simulink model "ThurstCalculation_Part1"  (R2017b)
settings: Solver=ode2  StartTime=0.0  StopTime=10  FixedStep=1/100  RelTol=1e-3  EnableMultiTasking=on
settings Model: Creator=dsde009  LastModifiedBy=Danyck
settings SolverCC: AlgebraicLoopSolver=LineSearch
settings DataIOCC: LimitDataPoints=on  SaveFormat=Array  SignalLoggingSaveFormat=ModelDataLogs  SignalLoggingName=SPE_DataLog
settings OptimizationCC: ExpressionDepthLimit=2147483647  InitFltsAndDblsToZero=on  LifeSpan=inf
settings DebuggingCC: ReadBeforeWriteMsg=DisableAll  WriteAfterWriteMsg=DisableAll  WriteAfterReadMsg=DisableAll  AlgebraicLoopMsg=none  SaveWithDisabledLinksMsg=none  UnderspecifiedInitializationDetection=Classic  MergeDetectMultiDrivingBlocksExec=none  MultiTaskDSMMsg=warning  MultiTaskCondExecSysMsg=none  ParameterPrecisionLossMsg=none  StateNameClashWarn=warning  SFUnexpectedBacktrackingDiag=warning  SFNoUnconditionalDefaultTransitionDiag=warning  SFExecutionAtInitializationDiag=none
settings HardwareCC: ProdBitPerPointer=32  ProdBitPerSizeT=32  ProdBitPerPtrDiffT=32  ProdLargestAtomicFloat=None  ProdIntDivRoundTo=Undefined  ProdEndianess=Unspecified  ProdWordSize=32  ProdHWDeviceType=32-bit Generic
settings ModelReferenceCC: UpdateModelReferenceTargets=IfOutOfDate  PropagateSignalLabelsOutOfModel=off
settings SFSimCC: SFSimEcho=off
settings CodeAppCC: StateflowObjectComments=on
settings GRTTargetCC: TargetLangStandard=C89/C90 (ANSI)  GeneratePreprocessorConditionals=Disable all  CombineOutputUpdateFcns=off  GRTInterface=on
settings ConfigComp: CovMetricSettings=dw  CovHtmlReporting=on  CovSaveCumulativeToWorkspaceVar=on  CovSaveSingleToWorkspaceVar=on  CovExternalEMLEnable=off  CovSFcnEnable=off

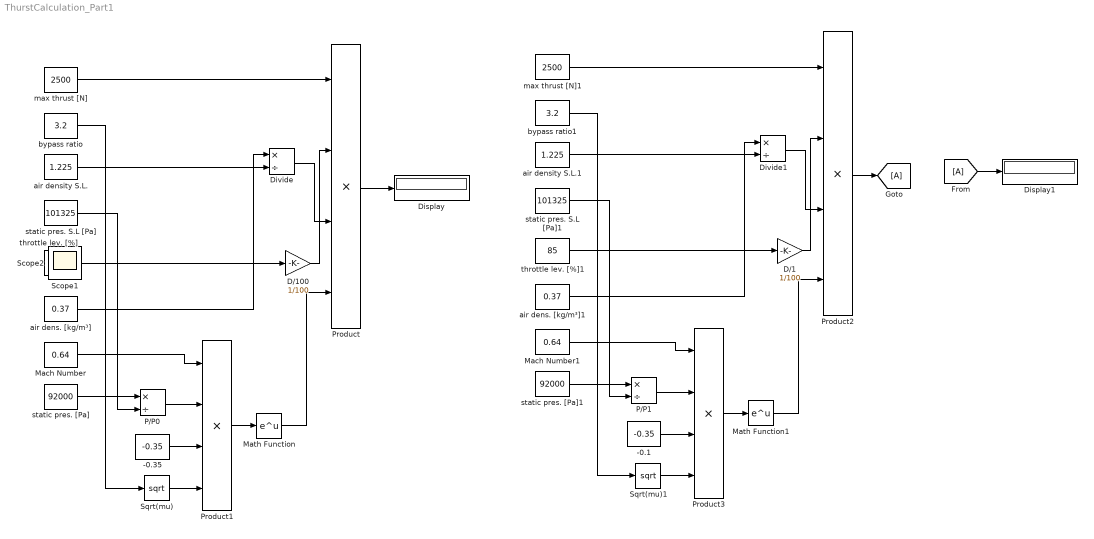
== system ThurstCalculation_Part1 ==
  -0.1 : Constant  Value=-0.35
  -0.35 : Constant  Value=-0.35
  D/1 : Gain  Gain=1/100
  D/100 : Gain  Gain=1/100
  Display : Display
  Display1 : Display
  Divide : Product  Inputs=*/
  Divide1 : Product  Inputs=*/
  Mach Number : Constant  Value=0.64
  Mach Number1 : Constant  Value=0.64
  Math Function : Math  SaturateOnIntegerOverflow=on
  Math Function1 : Math  SaturateOnIntegerOverflow=on
  P/P0 : Product  Inputs=*/
  P/P1 : Product  Inputs=*/
  Product{,1..3} (4 alike) : Product  Inputs=4
  Sqrt(mu) : Sqrt  SaturateOnIntegerOverflow=on
  Sqrt(mu)1 : Sqrt  SaturateOnIntegerOverflow=on
  air dens. [kg/m³] : Constant  Value=0.37
  air dens. [kg/m³]1 : Constant  Value=0.37
  air density S.L. : Constant  Value=1.225
  air density S.L.1 : Constant  Value=1.225
  bypass ratio : Constant  Value=3.2
  bypass ratio1 : Constant  Value=3.2
  max thrust [N] : Constant  Value=2500
  max thrust [N]1 : Constant  Value=2500
  static pres. S.L [Pa] : Constant  Value=101325
  static pres. S.L [Pa]1 : Constant  Value=101325
  static pres. [Pa] : Constant  Value=92000
  static pres. [Pa]1 : Constant  Value=92000
  throttle lev. [%] : Constant  Value=85
  throttle lev. [%]1 : Constant  Value=85
  Scope1 : Scope
  Scope2 : Scope
  wires:
  max thrust [N]/1 -> Product/1
  throttle lev. [%]/1 -> D/100/1
  D/100/1 -> Product/2
  air density S.L./1 -> Divide/2
  air dens. [kg/m³]/1 -> Divide/1
  Divide/1 -> Product/3
  static pres. [Pa]/1 -> P/P0/1
  static pres. S.L [Pa]/1 -> P/P0/2
  P/P0/1 -> Product1/2
  Mach Number/1 -> Product1/1
  -0.35/1 -> Product1/3
  bypass ratio/1 -> Sqrt(mu)/1
  Sqrt(mu)/1 -> Product1/4
  Product1/1 -> Math Function/1
  Math Function/1 -> Product/4
  Product/1 -> Display/1
  -0.1/1 -> Product3/3
  P/P1/1 -> Product3/2
  static pres. [Pa]1/1 -> P/P1/1
  air dens. [kg/m³]1/1 -> Divide1/1
  D/1/1 -> Product2/2
  Divide1/1 -> Product2/3
  max thrust [N]1/1 -> Product2/1
  Mach Number1/1 -> Product3/1
  Product3/1 -> Math Function1/1
  Math Function1/1 -> Product2/4
  Product2/1 -> [A]
  Sqrt(mu)1/1 -> Product3/4
  bypass ratio1/1 -> Sqrt(mu)1/1
  static pres. S.L [Pa]1/1 -> P/P1/2
  throttle lev. [%]1/1 -> D/1/1
  air density S.L.1/1 -> Divide1/2
  [A] -> Display1/1
